simulink model "orbitGuidance_LVLH"  (R2018a)
settings: Solver=VariableStepAuto  StartTime=0.0  StopTime=simDuration  RelTol=1e-3
values from neighbouring files (symbols this model uses):
  mu = 39.86004418*10^13    (= 398600441800000)    [simulinkLauncher.m]
  timestep = 1    [simulinkLauncher.m]
  v0Chaser = [7783 0 0]    [simulinkLauncher.m]
  v0Target = [7784 0 0]    [simulinkLauncher.m]
  x0Chaser = [0 6578e3 0]    [simulinkLauncher.m]
  x0Target = [0 6578e3 0]    [simulinkLauncher.m]
libraries: dspmtrx3 x21
settings Model: Creator=Yves-Marie  LastModifiedBy=Yves-Marie

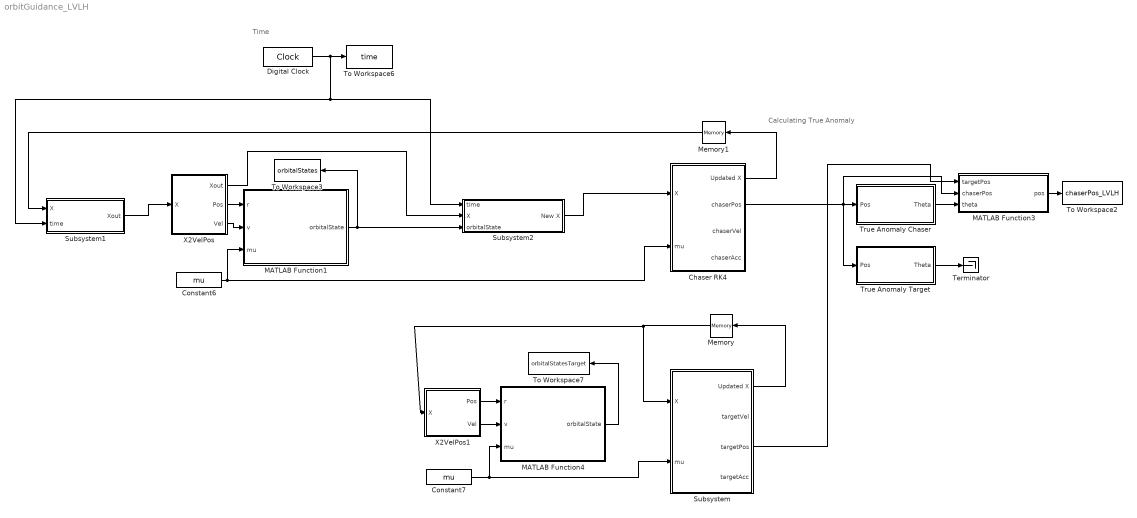
== system orbitGuidance_LVLH ==
  note: Time
  note: Calculating True Anomaly
  Chaser RK4 : Subsystem
  Constant6 : Constant  Value=mu
  Constant7 : Constant  Value=mu
  Digital Clock : DigitalClock
  MATLAB Function1 : MATLAB Function  TreatAsAtomicUnit=on
  MATLAB Function3 : MATLAB Function  TreatAsAtomicUnit=on
  MATLAB Function4 : MATLAB Function  TreatAsAtomicUnit=on
  Memory : Memory  InitialCondition=[x0Target;v0Target]  InheritSampleTime=on
  Memory1 : Memory  InitialCondition=[x0Chaser;v0Chaser]  InheritSampleTime=on
  Subsystem : Subsystem
  Subsystem1 : Subsystem
  Subsystem2 : Subsystem
  Terminator : Terminator
  To Workspace2 : ToWorkspace  VariableName=chaserPos_LVLH  SampleTime=-1
      settings: Save2DSignal=2-D array (concatenate along first dimension)
  To Workspace3 : ToWorkspace  VariableName=orbitalStates  SampleTime=-1
      settings: Save2DSignal=2-D array (concatenate along first dimension)
  To Workspace6 : ToWorkspace  VariableName=time  SampleTime=-1
      settings: Save2DSignal=2-D array (concatenate along first dimension)
  To Workspace7 : ToWorkspace  VariableName=orbitalStatesTarget  SampleTime=-1
      settings: Save2DSignal=2-D array (concatenate along first dimension)
  True Anomaly Chaser : Subsystem
  True Anomaly Target : Subsystem
  X2VelPos : Subsystem
  X2VelPos1 : Subsystem
  wires:
  MATLAB Function1/1(orbitalState) -> Subsystem2/3(orbitalState), To Workspace3/1
  Constant6/1 -> MATLAB Function1/3(mu), Chaser RK4/2(mu)
  Digital Clock/1 -> Subsystem2/1(time), Subsystem1/2(time), To Workspace6/1
  True Anomaly Chaser/1(Theta) -> MATLAB Function3/3(theta)
  MATLAB Function3/1(pos) -> To Workspace2/1
  Chaser RK4/2(chaserPos) -> MATLAB Function3/2(chaserPos), True Anomaly Target/1(Pos), True Anomaly Chaser/1(Pos)
  Constant7/1 -> MATLAB Function4/3(mu), Subsystem/2(mu)
  MATLAB Function4/1(orbitalState) -> To Workspace7/1
  True Anomaly Target/1(Theta) -> Terminator/1
  Subsystem/3(targetPos) -> MATLAB Function3/1(targetPos)
  X2VelPos/2(Pos) -> MATLAB Function1/1(r)
  X2VelPos/3(Vel) -> MATLAB Function1/2(v)
  Memory1/1 -> Subsystem1/1(X)
  X2VelPos1/1(Pos) -> MATLAB Function4/1(r)
  X2VelPos1/2(Vel) -> MATLAB Function4/2(v)
  Subsystem/1(Updated X) -> Memory/1
  Memory/1 -> Subsystem/1(X), X2VelPos1/1(X)
  Chaser RK4/1(Updated X) -> Memory1/1
  Subsystem1/1(Xout) -> X2VelPos/1(X)
  X2VelPos/1(Xout) -> Subsystem2/2(X)
  Subsystem2/1(New X) -> Chaser RK4/1(X)

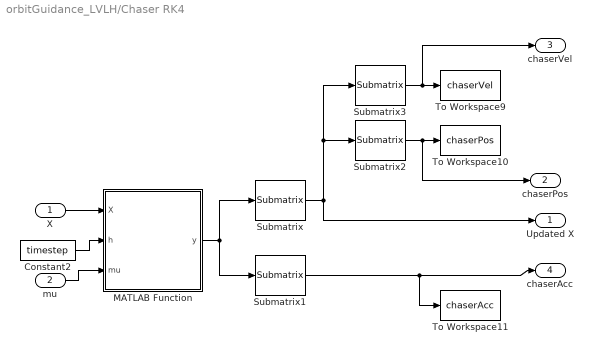
== system orbitGuidance_LVLH/Chaser RK4 ==
  X : Inport
  mu : Inport  Port=2
  Constant2 : Constant  Value=timestep
  MATLAB Function : MATLAB Function  TreatAsAtomicUnit=on
  Submatrix : dspmtrx3/Submatrix  RowSpan=Range of rows  RowStartMode=First  RowStartIndex=1  RowEndMode=Index  RowEndIndex=2  ColSpan=All columns  ColStartMode=First  ColStartIndex=1  ColEndMode=Last  ColEndIndex=1
  Submatrix1 : dspmtrx3/Submatrix  RowSpan=One row  RowStartMode=Last  RowStartIndex=1  RowEndMode=Index  RowEndIndex=2  ColSpan=All columns  ColStartMode=First  ColStartIndex=1  ColEndMode=Last  ColEndIndex=1
  Submatrix2 : dspmtrx3/Submatrix  RowSpan=One row  RowStartMode=First  RowStartIndex=1  RowEndMode=Index  RowEndIndex=2  ColSpan=All columns  ColStartMode=First  ColStartIndex=1  ColEndMode=Last  ColEndIndex=1
  Submatrix3 : dspmtrx3/Submatrix  RowSpan=One row  RowStartMode=Last  RowStartIndex=1  RowEndMode=Index  RowEndIndex=2  ColSpan=All columns  ColStartMode=First  ColStartIndex=1  ColEndMode=Last  ColEndIndex=1
  To Workspace10 : ToWorkspace  VariableName=chaserPos  SampleTime=-1
      settings: Save2DSignal=2-D array (concatenate along first dimension)
  To Workspace11 : ToWorkspace  VariableName=chaserAcc  SampleTime=-1
      settings: Save2DSignal=2-D array (concatenate along first dimension)
  To Workspace9 : ToWorkspace  VariableName=chaserVel  SampleTime=-1
      settings: Save2DSignal=2-D array (concatenate along first dimension)
  Updated X : Outport
  chaserPos : Outport  Port=2
  chaserVel : Outport  Port=3
  chaserAcc : Outport  Port=4
  wires:
  Submatrix2/1 -> chaserPos/1, To Workspace10/1
  MATLAB Function/1(y) -> Submatrix1/1, Submatrix/1
  Submatrix/1 -> Updated X/1, Submatrix3/1, Submatrix2/1
  Constant2/1 -> MATLAB Function/2(h)
  Submatrix1/1 -> To Workspace11/1, chaserAcc/1
  mu/1 -> MATLAB Function/3(mu)
  Submatrix3/1 -> chaserVel/1, To Workspace9/1
  X/1 -> MATLAB Function/1(X)

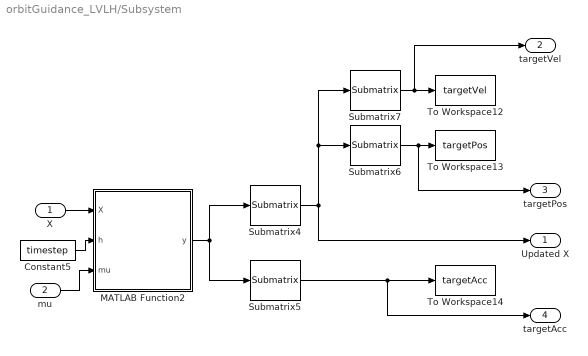
== system orbitGuidance_LVLH/Subsystem ==
  X : Inport
  mu : Inport  Port=2
  Constant5 : Constant  Value=timestep
  MATLAB Function2 : MATLAB Function  TreatAsAtomicUnit=on
  Submatrix4 : dspmtrx3/Submatrix  RowSpan=Range of rows  RowStartMode=First  RowStartIndex=1  RowEndMode=Index  RowEndIndex=2  ColSpan=All columns  ColStartMode=First  ColStartIndex=1  ColEndMode=Last  ColEndIndex=1
  Submatrix5 : dspmtrx3/Submatrix  RowSpan=One row  RowStartMode=Last  RowStartIndex=1  RowEndMode=Index  RowEndIndex=2  ColSpan=All columns  ColStartMode=First  ColStartIndex=1  ColEndMode=Last  ColEndIndex=1
  Submatrix6 : dspmtrx3/Submatrix  RowSpan=One row  RowStartMode=First  RowStartIndex=1  RowEndMode=Index  RowEndIndex=2  ColSpan=All columns  ColStartMode=First  ColStartIndex=1  ColEndMode=Last  ColEndIndex=1
  Submatrix7 : dspmtrx3/Submatrix  RowSpan=One row  RowStartMode=Last  RowStartIndex=1  RowEndMode=Index  RowEndIndex=2  ColSpan=All columns  ColStartMode=First  ColStartIndex=1  ColEndMode=Last  ColEndIndex=1
  To Workspace12 : ToWorkspace  VariableName=targetVel  SampleTime=-1
      settings: Save2DSignal=2-D array (concatenate along first dimension)
  To Workspace13 : ToWorkspace  VariableName=targetPos  SampleTime=-1
      settings: Save2DSignal=2-D array (concatenate along first dimension)
  To Workspace14 : ToWorkspace  VariableName=targetAcc  SampleTime=-1
      settings: Save2DSignal=2-D array (concatenate along first dimension)
  Updated X : Outport
  targetVel : Outport  Port=2
  targetPos : Outport  Port=3
  targetAcc : Outport  Port=4
  wires:
  Submatrix5/1 -> targetAcc/1, To Workspace14/1
  Submatrix7/1 -> targetVel/1, To Workspace12/1
  Submatrix4/1 -> Updated X/1, Submatrix7/1, Submatrix6/1
  Submatrix6/1 -> targetPos/1, To Workspace13/1
  Constant5/1 -> MATLAB Function2/2(h)
  MATLAB Function2/1(y) -> Submatrix5/1, Submatrix4/1
  X/1 -> MATLAB Function2/1(X)
  mu/1 -> MATLAB Function2/3(mu)

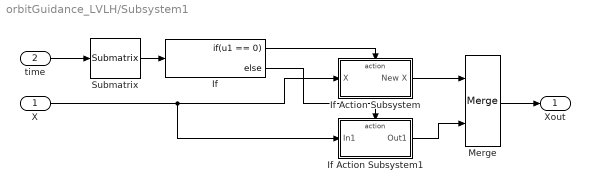
== system orbitGuidance_LVLH/Subsystem1 ==
  X : Inport
  time : Inport  Port=2
  If : If  IfExpression=u1 == 0
  If Action Subsystem : Subsystem  TreatAsAtomicUnit=on
  If Action Subsystem1 : Subsystem  TreatAsAtomicUnit=on
  Merge : Merge  InitialOutput=[0 0 0;0 0 0]
  Submatrix : dspmtrx3/Submatrix  RowSpan=One row  RowStartMode=Last  RowStartIndex=1  RowEndMode=Last  RowEndIndex=1  ColSpan=One column  ColStartMode=First  ColStartIndex=1  ColEndMode=Last  ColEndIndex=1
  Xout : Outport
  wires:
  time/1 -> Submatrix/1
  Submatrix/1 -> If/1
  Merge/1 -> Xout/1
  If/1 -> If Action Subsystem/Action
  If Action Subsystem/1(New X) -> Merge/1
  If/2 -> If Action Subsystem1/Action
  X/1 -> If Action Subsystem/1(X), If Action Subsystem1/1(In1)
  If Action Subsystem1/1(Out1) -> Merge/2

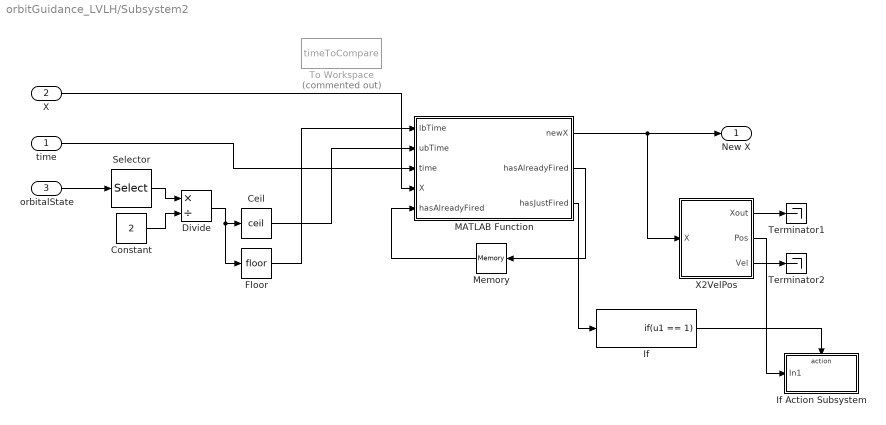
== system orbitGuidance_LVLH/Subsystem2 ==
  time : Inport
  X : Inport  Port=2
  orbitalState : Inport  Port=3
  Ceil : Rounding  Operator=ceil
  Constant : Constant  Value=2
  Divide : Product  Inputs=*/
  Floor : Rounding
  If : If  IfExpression=u1 == 1  ShowElse=off
  If Action Subsystem : Subsystem  TreatAsAtomicUnit=on
  MATLAB Function : MATLAB Function  TreatAsAtomicUnit=on
  Memory : Memory  InheritSampleTime=on  LinearizeMemory=on
  Selector : Selector  InputPortWidth=11  IndexOptions=Index vector (dialog)  Indices=[11]  OutputSizes=1
  Terminator1 : Terminator
  Terminator2 : Terminator
  To Workspace : ToWorkspace  Commented=on  VariableName=timeToCompare  SampleTime=-1
      settings: Save2DSignal=2-D array (concatenate along first dimension)
  X2VelPos : Subsystem
  New X : Outport
  wires:
  Selector/1 -> Divide/1
  Constant/1 -> Divide/2
  orbitalState/1 -> Selector/1
  Divide/1 -> Floor/1, Ceil/1
  MATLAB Function/1(newX) -> X2VelPos/1(X), New X/1
  time/1 -> MATLAB Function/3(time)
  X/1 -> MATLAB Function/4(X)
  Memory/1 -> MATLAB Function/5("hasAlreadyFired ")
  MATLAB Function/2(hasAlreadyFired) -> Memory/1
  MATLAB Function/3(hasJustFired) -> If/1
  If/1 -> If Action Subsystem/Action
  X2VelPos/2(Pos) -> If Action Subsystem/1(In1)
  X2VelPos/1(Xout) -> Terminator1/1
  X2VelPos/3(Vel) -> Terminator2/1
  Ceil/1 -> MATLAB Function/2(ubTime)
  Floor/1 -> MATLAB Function/1(lbTime)

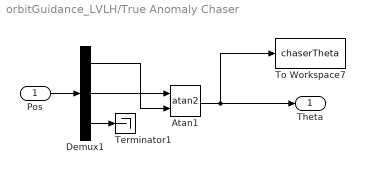
== system orbitGuidance_LVLH/True Anomaly Chaser ==
  Pos : Inport
  Atan1 : Trigonometry  Operator=atan2  OutputSignalType=real
  Demux1 : Demux  Outputs=3
  Terminator1 : Terminator
  To Workspace7 : ToWorkspace  VariableName=chaserTheta  SampleTime=-1
      settings: Save2DSignal=2-D array (concatenate along first dimension)
  Theta : Outport
  wires:
  Pos/1 -> Demux1/1
  Demux1/2 -> Atan1/1
  Demux1/1 -> Atan1/2
  Demux1/3 -> Terminator1/1
  Atan1/1 -> Theta/1, To Workspace7/1

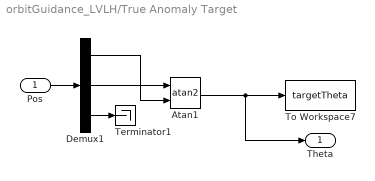
== system orbitGuidance_LVLH/True Anomaly Target ==
  Pos : Inport
  Atan1 : Trigonometry  Operator=atan2  OutputSignalType=real
  Demux1 : Demux  Outputs=3
  Terminator1 : Terminator
  To Workspace7 : ToWorkspace  VariableName=targetTheta  SampleTime=-1
      settings: Save2DSignal=2-D array (concatenate along first dimension)
  Theta : Outport
  wires:
  Demux1/3 -> Terminator1/1
  Demux1/1 -> Atan1/2
  Demux1/2 -> Atan1/1
  Pos/1 -> Demux1/1
  Atan1/1 -> To Workspace7/1, Theta/1

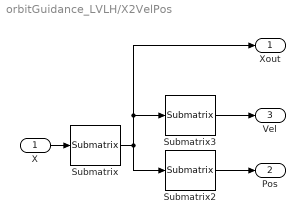
== system orbitGuidance_LVLH/X2VelPos ==
  X : Inport
  Submatrix : dspmtrx3/Submatrix  RowSpan=Range of rows  RowStartMode=First  RowStartIndex=1  RowEndMode=Index  RowEndIndex=2  ColSpan=All columns  ColStartMode=First  ColStartIndex=1  ColEndMode=Last  ColEndIndex=1
  Submatrix2 : dspmtrx3/Submatrix  RowSpan=One row  RowStartMode=First  RowStartIndex=1  RowEndMode=Index  RowEndIndex=2  ColSpan=All columns  ColStartMode=First  ColStartIndex=1  ColEndMode=Last  ColEndIndex=1
  Submatrix3 : dspmtrx3/Submatrix  RowSpan=One row  RowStartMode=Last  RowStartIndex=1  RowEndMode=Index  RowEndIndex=2  ColSpan=All columns  ColStartMode=First  ColStartIndex=1  ColEndMode=Last  ColEndIndex=1
  Xout : Outport
  Pos : Outport  Port=2
  Vel : Outport  Port=3
  wires:
  Submatrix/1 -> Submatrix2/1, Xout/1, Submatrix3/1
  X/1 -> Submatrix/1
  Submatrix3/1 -> Vel/1
  Submatrix2/1 -> Pos/1

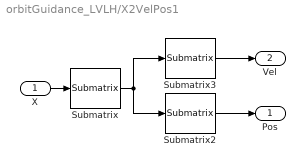
== system orbitGuidance_LVLH/X2VelPos1 ==
  X : Inport
  Submatrix : dspmtrx3/Submatrix  RowSpan=Range of rows  RowStartMode=First  RowStartIndex=1  RowEndMode=Index  RowEndIndex=2  ColSpan=All columns  ColStartMode=First  ColStartIndex=1  ColEndMode=Last  ColEndIndex=1
  Submatrix2 : dspmtrx3/Submatrix  RowSpan=One row  RowStartMode=First  RowStartIndex=1  RowEndMode=Index  RowEndIndex=2  ColSpan=All columns  ColStartMode=First  ColStartIndex=1  ColEndMode=Last  ColEndIndex=1
  Submatrix3 : dspmtrx3/Submatrix  RowSpan=One row  RowStartMode=Last  RowStartIndex=1  RowEndMode=Index  RowEndIndex=2  ColSpan=All columns  ColStartMode=First  ColStartIndex=1  ColEndMode=Last  ColEndIndex=1
  Pos : Outport
  Vel : Outport  Port=2
  wires:
  Submatrix2/1 -> Pos/1
  Submatrix3/1 -> Vel/1
  X/1 -> Submatrix/1
  Submatrix/1 -> Submatrix3/1, Submatrix2/1

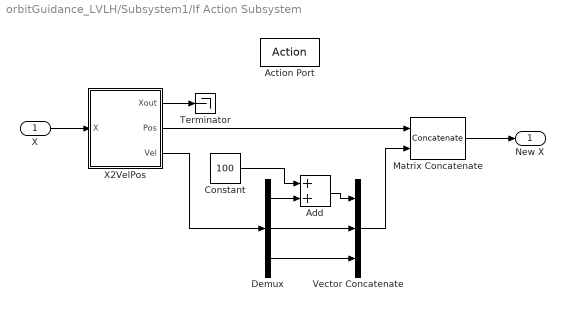
== system orbitGuidance_LVLH/Subsystem1/If Action Subsystem ==
  X : Inport
  Action Port : ActionPort  ActionType=then
  Add : Sum
  Constant : Constant  Value=100
  Demux : Demux  Outputs=3
  Matrix Concatenate : Concatenate  Mode=Multidimensional array
  Terminator : Terminator
  Vector Concatenate : Concatenate  NumInputs=3  Mode=Multidimensional array  ConcatenateDimension=2
  X2VelPos : Subsystem
  New X : Outport
  wires:
  Matrix Concatenate/1 -> New X/1
  X2VelPos/3(Vel) -> Demux/1
  X/1 -> X2VelPos/1(X)
  Demux/1 -> Add/2
  Constant/1 -> Add/1
  Demux/2 -> Vector Concatenate/2
  Vector Concatenate/1 -> Matrix Concatenate/2
  Demux/3 -> Vector Concatenate/3
  X2VelPos/2(Pos) -> Matrix Concatenate/1
  Add/1 -> Vector Concatenate/1
  X2VelPos/1(Xout) -> Terminator/1

== system orbitGuidance_LVLH/Subsystem1/If Action Subsystem1 ==
  In1 : Inport
  Action Port : ActionPort  ActionType=else
  Out1 : Outport
  wires:
  In1/1 -> Out1/1

== system orbitGuidance_LVLH/Subsystem2/If Action Subsystem ==
  In1 : Inport
  Action Port : ActionPort  ActionType=then
  To Workspace : ToWorkspace  VariableName=chaserFiringPos  SampleTime=-1
      settings: Save2DSignal=2-D array (concatenate along first dimension)
  wires:
  In1/1 -> To Workspace/1

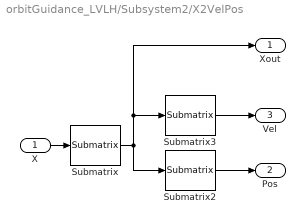
== system orbitGuidance_LVLH/Subsystem2/X2VelPos ==
  X : Inport
  Submatrix : dspmtrx3/Submatrix  RowSpan=Range of rows  RowStartMode=First  RowStartIndex=1  RowEndMode=Index  RowEndIndex=2  ColSpan=All columns  ColStartMode=First  ColStartIndex=1  ColEndMode=Last  ColEndIndex=1
  Submatrix2 : dspmtrx3/Submatrix  RowSpan=One row  RowStartMode=First  RowStartIndex=1  RowEndMode=Index  RowEndIndex=2  ColSpan=All columns  ColStartMode=First  ColStartIndex=1  ColEndMode=Last  ColEndIndex=1
  Submatrix3 : dspmtrx3/Submatrix  RowSpan=One row  RowStartMode=Last  RowStartIndex=1  RowEndMode=Index  RowEndIndex=2  ColSpan=All columns  ColStartMode=First  ColStartIndex=1  ColEndMode=Last  ColEndIndex=1
  Xout : Outport
  Pos : Outport  Port=2
  Vel : Outport  Port=3
  wires:
  Submatrix/1 -> Submatrix2/1, Xout/1, Submatrix3/1
  X/1 -> Submatrix/1
  Submatrix3/1 -> Vel/1
  Submatrix2/1 -> Pos/1

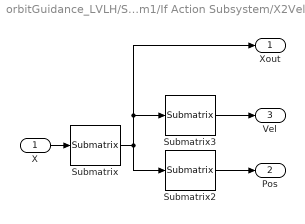
== system orbitGuidance_LVLH/Subsystem1/If Action Subsystem/X2VelPos ==
  X : Inport
  Submatrix : dspmtrx3/Submatrix  RowSpan=Range of rows  RowStartMode=First  RowStartIndex=1  RowEndMode=Index  RowEndIndex=2  ColSpan=All columns  ColStartMode=First  ColStartIndex=1  ColEndMode=Last  ColEndIndex=1
  Submatrix2 : dspmtrx3/Submatrix  RowSpan=One row  RowStartMode=First  RowStartIndex=1  RowEndMode=Index  RowEndIndex=2  ColSpan=All columns  ColStartMode=First  ColStartIndex=1  ColEndMode=Last  ColEndIndex=1
  Submatrix3 : dspmtrx3/Submatrix  RowSpan=One row  RowStartMode=Last  RowStartIndex=1  RowEndMode=Index  RowEndIndex=2  ColSpan=All columns  ColStartMode=First  ColStartIndex=1  ColEndMode=Last  ColEndIndex=1
  Xout : Outport
  Pos : Outport  Port=2
  Vel : Outport  Port=3
  wires:
  Submatrix/1 -> Submatrix2/1, Xout/1, Submatrix3/1
  X/1 -> Submatrix/1
  Submatrix3/1 -> Vel/1
  Submatrix2/1 -> Pos/1

== matlab function orbitGuidance_LVLH/MATLAB Function1 ==
  data: r input; orbitalState output; v input; mu input
function orbitalState = rv2Orbit(r,v,mu)
    % From the 3D position vector 'r' of the spacecraft in meters, its
    % velocity vector in m/s 'v' and the standard gravitational constant of
    % the orbited planet, returns the orbital parameters of the
    % spacecraft's orbit.

    vNorm = norm(v);
    rNorm = norm(r);
    a = rNorm*mu / (2*mu - rNorm*vNorm*vNorm);
    T = 2*pi*sqrt(a^3/mu);
    h = cross(r,v);
    eVec = cross(v,h)/mu - r/rNorm;
    e = norm(eVec);
    p = a*(1-e*e);
    b = sqrt(p*a);
    c = a*e;
    ra = a+c;
    rp = 2*a - ra;
    
    ascNVec = cross([1;0;0], h);
    i = (pi/2 - acos(h(2)/norm(ascNVec))) * 180/pi;
    lAscN = acos(ascNVec(1)/norm(ascNVec));
    if(ascNVec(3) >= 0)
        lAscN = ClampAngle(0,pi,lAscN);
    else
        lAscN = ClampAngle(pi,2*pi,lAscN);
    end
    lAscN = (pi/2-lAscN) * 180/pi;
    
    omega = 0;
    if(norm(ascNVec)*norm(eVec) ~= 0)
        omega = acos(dot(ascNVec,eVec)/norm(ascNVec)*norm(eVec)) * 180/pi;
    end
    orbitalState = [ra,rp,e,p,a,b,c,i,lAscN,omega,T];
end

== matlab function orbitGuidance_LVLH/Chaser RK4/MATLAB Function ==
  data: X input size=[2;3]; y output double size=[3;3]; h input double size=1; mu input double size=1
function y = rk4Step(X,h,mu)
    % Performs one step of the Runge-Kutta 4th order propagator
    % X is the state matrix
    % h is the timestep
    k1 = GetKRKV(X,mu);        % k1
    k2 = GetKRKV(X+k1*h/2,mu); % k2
    k3 = GetKRKV(X+k2*h/2,mu); % k3
    k4 = GetKRKV(X+k3*h,mu);   % k2
    
    X = X + (h/6)*(k1 + 2*k2 + 2*k3 + k4);
    y = [X;k1(2,:)];
end

== matlab function orbitGuidance_LVLH/Subsystem/MATLAB Function2 ==
  data: X input size=[2;3]; y output double size=[3;3]; h input double size=1; mu input double size=1
function y = rk4Step(X,h,mu)
    coder.extrinsic('exist');
    % Performs one step of the Runge-Kutta 4th order propagator
    % X is the state matrix
    % h is the timestep
    k1 = GetKRKV(X,mu);        % k1
    k2 = GetKRKV(X+k1*h/2,mu); % k2
    k3 = GetKRKV(X+k2*h/2,mu); % k3
    k4 = GetKRKV(X+k3*h,mu);   % k2
    
    X = X + (h/6)*(k1 + 2*k2 + 2*k3 + k4);
    y = [X;k1(2,:)];
end

== matlab function orbitGuidance_LVLH/MATLAB Function3 ==
  data: targetPos input; chaserPos input; theta input; pos output
function pos = LVLH(targetPos,chaserPos,theta)
    pos = (chaserPos-targetPos)*[sin(theta) cos(theta) 0; cos(theta) -sin(theta) 0; 0 0 1];
end

== matlab function orbitGuidance_LVLH/MATLAB Function4 ==
  data: r input; orbitalState output; v input; mu input
function orbitalState = rv2Orbit(r,v,mu)
    % From the 3D position vector 'r' of the spacecraft in meters, its
    % velocity vector in m/s 'v' and the standard gravitational constant of
    % the orbited planet, returns the orbital parameters of the
    % spacecraft's orbit.

    vNorm = norm(v);
    rNorm = norm(r);
    a = rNorm*mu / (2*mu - rNorm*vNorm*vNorm);
    T = 2*pi*sqrt(a^3/mu);
    h = cross(r,v);
    eVec = cross(v,h)/mu - r/rNorm;
    e = norm(eVec);
    p = a*(1-e*e);
    b = sqrt(p*a);
    c = a*e;
    ra = a+c;
    rp = 2*a - ra;
    
    ascNVec = cross([1;0;0], h);
    i = (pi/2 - acos(h(2)/norm(ascNVec))) * 180/pi;
    lAscN = acos(ascNVec(1)/norm(ascNVec));
    if(ascNVec(3) >= 0)
        lAscN = ClampAngle(0,pi,lAscN);
    else
        lAscN = ClampAngle(pi,2*pi,lAscN);
    end
    lAscN = (pi/2-lAscN) * 180/pi;
    
    omega = 0;
    if(norm(ascNVec)*norm(eVec) ~= 0)
        omega = acos(dot(ascNVec,eVec)/norm(ascNVec)*norm(eVec)) * 180/pi;
    end
    orbitalState = [ra,rp,e,p,a,b,c,i,lAscN,omega,T];
end

== matlab function orbitGuidance_LVLH/Subsystem2/MATLAB Function ==
  data: lbTime input; newX output; hasAlreadyFired output; ubTime input; time input; X input; hasAlreadyFired input; hasJustFired output
function [newX,hasAlreadyFired,hasJustFired] = fcn(lbTime, ubTime, time, X, hasAlreadyFired)
    if(lbTime <= time && ubTime >= time && hasAlreadyFired == 0)
        pos = X(1,:);
        vel = X(2,:);
        newVel = [vel(1)+100 vel(2) vel(3)];
        newX = [pos;newVel];
        hasAlreadyFired = 1;
        hasJustFired = 1;
    else
        newX = X;
        hasJustFired = 0;
        %hasAlreadyFired = hasAlreadyFired;
    end
end
